simulink subsystem "DemandEletricityPrice"  (R2022b)
settings: Solver=VariableStepAuto  StartTime=0.0  StopTime=10.0  RelTol=1e-3
settings Model: Creator=is123  LastModifiedBy=is123

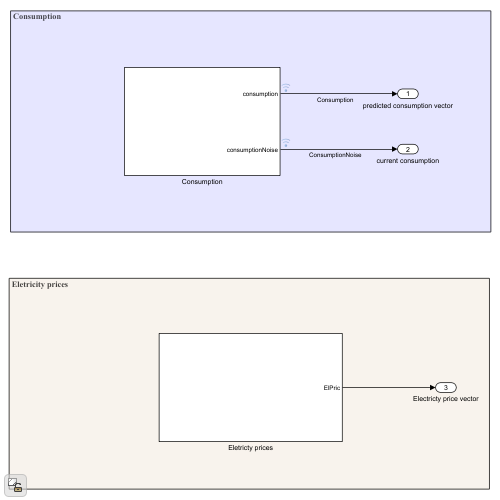
[thumbnail: Simulink's stored preview of the top-level diagram]
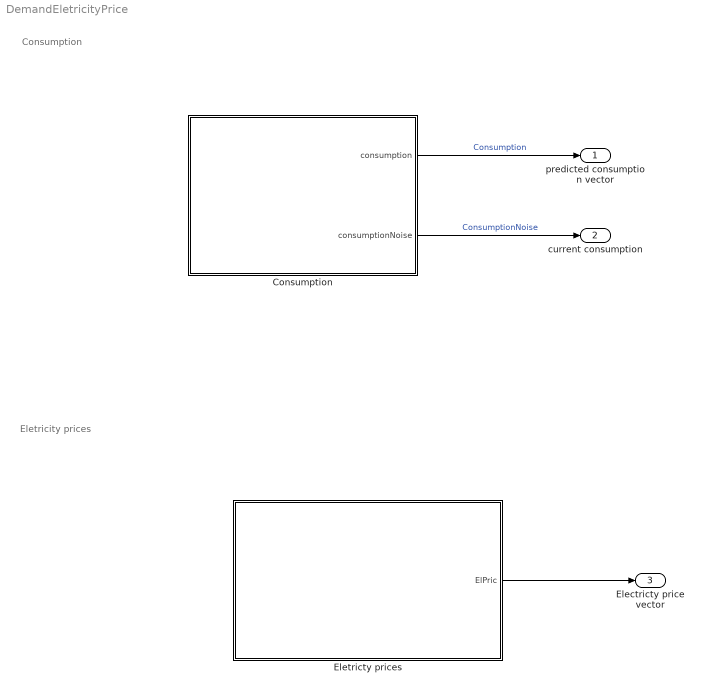
== system DemandEletricityPrice ==
  note: Consumption
  note: Eletricity prices
  Consumption : Subsystem
  Eletricty prices : Subsystem
  predicted consumption vector : Outport
  current consumption : Outport  Port=2
  Electricty price vector : Outport  Port=3
  wires:
  Eletricty prices/1(ElPric) -> Electricty price vector/1
  Consumption/1(consumption) -> predicted consumption vector/1  "Consumption"
  Consumption/2(consumptionNoise) -> current consumption/1  "ConsumptionNoise"

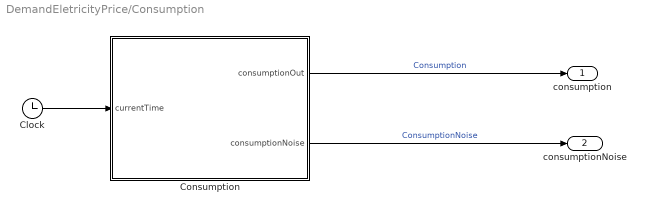
== system DemandEletricityPrice/Consumption ==
  Clock : Clock
  Consumption : MATLAB Function  TreatAsAtomicUnit=on  SystemSampleTime=3600/6
  consumption : Outport
  consumptionNoise : Outport  Port=2
  wires:
  Clock/1 -> Consumption/1(currentTime)
  Consumption/2(consumptionNoise) -> consumptionNoise/1  "ConsumptionNoise"
  Consumption/1(consumptionOut) -> consumption/1  "Consumption"

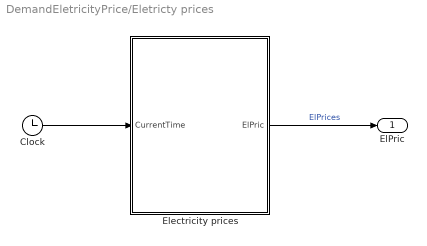
== system DemandEletricityPrice/Eletricty prices ==
  Clock : Clock
  Electricity prices : MATLAB Function  TreatAsAtomicUnit=on  SystemSampleTime=3600/6
  ElPric : Outport
  wires:
  Clock/1 -> Electricity prices/1(CurrentTime)
  Electricity prices/1(ElPric) -> ElPric/1  "ElPrices"

== matlab function DemandEletricityPrice/Consumption/Consumption ==
  data: currentTime input; consumptionOut output; consumptionNoise output
function [consumptionOut,consumptionNoise]  = consumption_simulink(currentTime)
%Getting the consumption for MPC and model 
c=scaled_standard_constants;
%Setting to use accelered time


%Giving the system the first 10 minuts to start up 
if currentTime <200 
    consumptionNoise=0;
    consumptionOut=zeros(c.Nc,1); 
else 

%Calling the consumption to get the consumptions needed 
[consumptionOutTemp,consumptionNoiseTemp]=consumption(currentTime); 

if c.disturbance==true
%For the model only the first consumption is neccesary! 
    consumptionNoise=consumptionNoiseTemp(1,1); 
    consumptionOut=consumptionOutTemp(1:c.Nc,1);
else  
    consumptionNoise=consumptionOutTemp(1,1);
    consumptionOut=consumptionOutTemp(1:c.Nc,1);
end 

end 
end

== matlab function DemandEletricityPrice/Eletricty prices/Electricity prices ==
  data: CurrentTime input; ElPric output
function ElPric = ElPrices(CurrentTime)
%loading in standard scaled constants 
c=scaled_standard_constants; 
%Giving the system 10 minuts: 
if CurrentTime <200 
    ElPric=zeros(c.Nc,1); 
else 

    %Calling matlab function to get the electricty price
    [ElPricTemp]=ElectrictyPrices(CurrentTime);
    ElPric=ElPricTemp;

end 

end
